simulink model "VSG"  (R2022a)
settings: Solver=ode23t  StartTime=0.0  StopTime=3  RelTol=1e-3
values from neighbouring files (symbols this model uses):
  C = 5600e-6    (= 0.0056)    [param.m]
  Cf = 35e-6    (= 3.5e-05)    [param.m]
  D = 3.24e4/w0    (= 103.132403124)    [param.m]
  E0 = 311    [param.m]
  fn = 50    [param.m]
  Ib = Sb/(sqrt(3)*Ub)    [param.m]
  J = 3.36    [param.m]
  Kf = 0.95e4/w0    (= 30.2394391875)    [param.m]
  Ki = 0.5*sqrt(3)*Sb/Ub    [param.m]
  Kq = (2500*6000)/(800e3*sqrt(3))    [param.m]
  L = 3e-3    (= 0.003)    [param.m]
  Pref = 170e3    (= 170000)    [param.m]
  R = 0.5    [param.m]
  Rc = 1e-3    (= 0.001)    [param.m]
  Rf = 0.05    [param.m]
  Sb = 800e3    (= 800000)    [param.m]
  Ts = 1/20e3    (= 5e-05)    [param.m]
  Ub = 6e3    (= 6000)    [param.m]
  Un = 380    [param.m]
  w0 = 2*pi*fn    (= 314.159265359)    [param.m]
libraries: spsIGBTDiodeLib x14, spsSeriesRLCBranchLib x9, slpidlib x7, spsDiodeLib x6, spsVoltageMeasurementLib x6, spsabctodq0Lib x4, spsThreePhaseVIMeasurementLib x3, eePowerMeasurement x2, simulink x2, spsDCVoltageSourceLib x1, spsGroundLib x1, spsPower3phInstantaneousLib x1
(part 1 of 2)
settings Model: Creator=Ziang Liu  LastModifiedBy=Ziang Liu

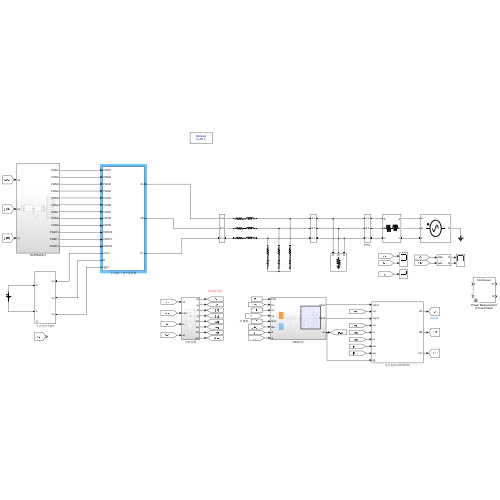
[thumbnail: Simulink's stored preview of the top-level diagram]
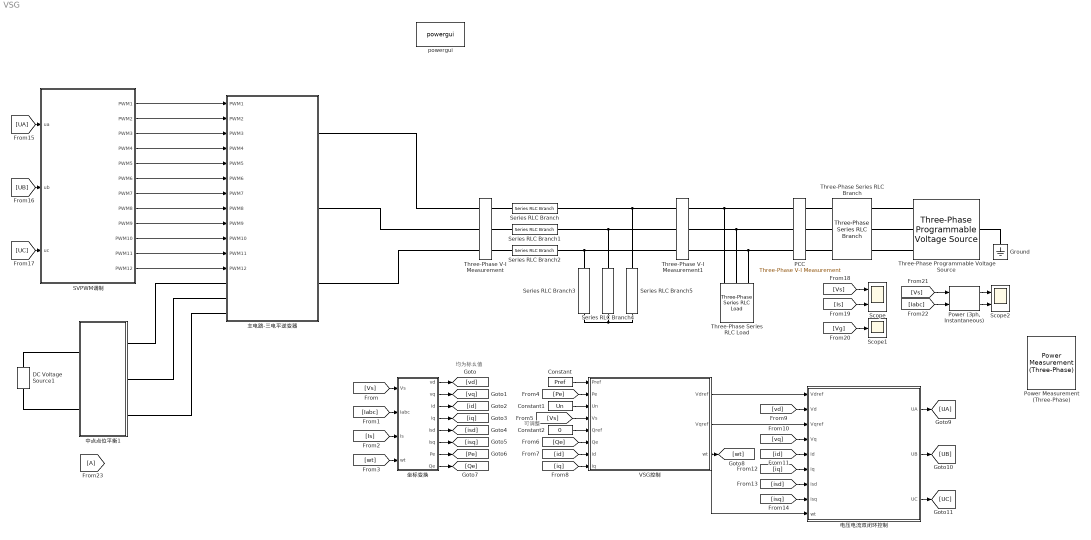
== system VSG ==
  note: 可调整
  note: 均为标幺值
  Constant : Constant  Value=Pref
  Constant1 : Constant  Value=Un
  Constant2 : Constant  Value=0
  DC Voltage Source1 : spsDCVoltageSourceLib/DC Voltage Source  Amplitude=1000  Measurements=None
  From23 : From
  Ground : spsGroundLib/Ground  LConnTagsString=a
  PCC : spsThreePhaseVIMeasurementLib/Three-Phase V-I Measurement  VoltageMeasurement=phase-to-ground  SetLabelV=on  LabelV=Vg  Vpu=off  VpuLL=off  CurrentMeasurement=no  SetLabelI=off  LabelI=Is  Ipu=off  Pbase=100e6  Vbase=500e3  OutputType=Complex  PhasorSimulation=off  PSBequivalent=0
  "Power (3ph, Instantaneous)" : spsPower3phInstantaneousLib/Power (3ph, Instantaneous)
  Power Measurement (Three-Phase) : eePowerMeasurement/Power Measurement (Three-Phase)  LabelModeActiveChoice=Continuous  F=60  K=[0 1 2 3]  Seq=Positive  Ts=0
      settings: SourceProductBaseCode=PS
  SVPWM调制 : Subsystem
  Scope : Scope  NumInputPorts=2
  Scope1 : Scope
  Scope2 : Scope  NumInputPorts=2
  Series RLC Branch : spsSeriesRLCBranchLib/Series RLC Branch  LConnTagsString=__new0  RConnTagsString=__new0  BranchType=RL  Resistance=Rf  Inductance=L  SetiL0=off  InitialCurrent=0  Capacitance=1e-6  Setx0=off  InitialVoltage=0  Measurements=None
  Series RLC Branch1 : spsSeriesRLCBranchLib/Series RLC Branch  LConnTagsString=__new0  RConnTagsString=__new0  BranchType=RL  Resistance=Rf  Inductance=L  SetiL0=off  InitialCurrent=0  Capacitance=1e-6  Setx0=off  InitialVoltage=0  Measurements=None
  Series RLC Branch2 : spsSeriesRLCBranchLib/Series RLC Branch  LConnTagsString=__new0  RConnTagsString=__new0  BranchType=RL  Resistance=Rf  Inductance=L  SetiL0=off  InitialCurrent=0  Capacitance=1e-6  Setx0=off  InitialVoltage=0  Measurements=None
  Series RLC Branch3 : spsSeriesRLCBranchLib/Series RLC Branch  LConnTagsString=__new0  RConnTagsString=__new0  BranchType=RC  Resistance=R  Inductance=L  SetiL0=off  InitialCurrent=0  Capacitance=Cf  Setx0=off  InitialVoltage=0  Measurements=None
  Series RLC Branch4 : spsSeriesRLCBranchLib/Series RLC Branch  LConnTagsString=__new0  RConnTagsString=__new0  BranchType=RC  Resistance=R  Inductance=L  SetiL0=off  InitialCurrent=0  Capacitance=Cf  Setx0=off  InitialVoltage=0  Measurements=None
  Series RLC Branch5 : spsSeriesRLCBranchLib/Series RLC Branch  LConnTagsString=__new0  RConnTagsString=__new0  BranchType=RC  Resistance=R  Inductance=L  SetiL0=off  InitialCurrent=0  Capacitance=Cf  Setx0=off  InitialVoltage=0  Measurements=None
  Three-Phase Programmable Voltage Source : spsThreePhaseProgrammableVoltageSourceLib/Three-Phase Programmable Voltage Source  PositiveSequence="[380  0 50]"  VariationEntity=Frequency  VariationType=Table of time-amplitude pairs  VariationTypeAlt=Step  VariationStep=-0.2  VariationRate=10  VariationMagnitude=0.3  VariationFrequency=2  VariationTiming=[1 2]  VariationPhaseA=off  Amplitudes=[1 0.8 1.2 1.0]  TimeValues=[0 0.1 0.15 0.2]  HarmonicGeneration=off  HarmonicA=[3 0.2 -25 0]  HarmonicB=[2 0.15 35 2]  Timing="[0.05  3]"  BusType=swing  Pref=0  Qref=0  Qmin=-inf  Qmax=inf
  Three-Phase Series RLC Branch : spsThreePhaseSeriesRLCBranchLib/Three-Phase Series RLC Branch  LConnTagsString=A|B|C  RConnTagsString=A|B|C  BranchType=RL  Resistance=0.06  Inductance=1.35e-3  Capacitance=1e-6  Measurements=None
  Three-Phase Series RLC Load : spsThreePhaseSeriesRLCLoadLib/Three-Phase Series RLC Load  LConnTagsString=A|B|C  Configuration=Y (grounded)  NominalVoltage=380  Vabc=[1e3 1e3 1e3]  Vabcp=[1e3 1e3 1e3]  NominalFrequency=50  UnbalancedPower=off  ActivePower=120e3  InductivePower=0  CapacitivePower=0  Pabc=[10e3 9e3 11e3]  QLabc=[100 90 110]  QCabc=[100 90 110]  Pabcp=[10e3 9e3 11e3]  QLabcp=[100 90 110]  QCabcp=[100 90 110]  Measurements=None  LoadType=constant Z
  Three-Phase V-I Measurement : spsThreePhaseVIMeasurementLib/Three-Phase V-I Measurement  VoltageMeasurement=no  SetLabelV=off  LabelV=Vabc  Vpu=off  VpuLL=off  CurrentMeasurement=yes  SetLabelI=on  LabelI=Iabc  Ipu=off  Pbase=100e6  Vbase=500e3  OutputType=Complex  PhasorSimulation=off  PSBequivalent=0
  Three-Phase V-I Measurement1 : spsThreePhaseVIMeasurementLib/Three-Phase V-I Measurement  VoltageMeasurement=phase-to-ground  SetLabelV=on  LabelV=Vs  Vpu=off  VpuLL=off  CurrentMeasurement=yes  SetLabelI=on  LabelI=Is  Ipu=off  Pbase=100e6  Vbase=500e3  OutputType=Complex  PhasorSimulation=off  PSBequivalent=0
  VSG控制 : Subsystem
  powergui : spspowerguiLib/powergui  Priority=1  SimulationMode=Discrete  SampleTime=1e-6  frequency=60  Iterations=50  frequencyindice=50  Pbase=100e6  ErrMax=1e-4  UnitsV=kV  UnitsW=MW  buscounter=0  FunctionMessages=off  echomessages=off  EnableUseOfTLC=off  CurrentSourceSwitches=off  DisableSnubberDevices=off  DisableRonSwitches=off  DisableVfSwitches=off  DisplayEquations=off  AutomaticDiscreteSolvers=off  SolverType=Tustin/Backward Euler (TBE)  Interpol=off  ExternalGateDelay=off  methode=off  Ts=100  x0status=blocks  SPID=on  SwTol=0  HookPort=off  NonlinearTolerance=1e-4  nMaxIteration=100  ContinueOnMaxIteration=off  RestoreLinks=warning  ResistiveCurrentMeasurement=off  Frange=[0:2:500]  Ylog=off  Xlog=on  ShowGrid=off  save=off  variable=ZData  structure=0  ZoomFFT=off  StartTime=0.0  cycles=1  DisplayStyle=1  fundamental=60  FreqAxis=off  MaxFrequency=1000  frequencyindicesteady=1  RmsSteady=1  display=off
  中点点位平衡1 : Subsystem  mask{Ln=2e-3, Kp1=20.73, Ki1=4.2, Kp2=5.5, Ki2=2.7}
      mask prompts: Ln "平衡电感Ln："; Kp1 "电压外环Kp1："; Ki1 "电压外环Ki1："; Kp2 "电流内环Kp2："; Ki2 "电流内环Ki2"
      mask DialogControl ParameterGroupVar Prompt: 参数
  主电路-三电平逆变器 : Subsystem  mask{Rc=1e-3, C=5600e-6}
      mask prompts: Rc "电容等效电阻Rc"; C "直流电容C:"
      mask DialogControl ParameterGroupVar Prompt: 参数
  坐标变换 : Subsystem
  电压电流双闭环控制 : Subsystem  mask{Kpu=6, Kiu=153.33, Kpi=4.2, Kii=0.323, wC=2*pi*fn*Cf*(Sb/(Ub^2)), wL=2*pi*fn*L*(Sb/(Ub^2))}
      mask prompts: Kpu "电压环比例系数Kpu:"; Kiu "电压环积分系数Kiu:"; Kpi "电流环比例系数Kpi:"; Kii "电流环v积分系数Kii:"; wC "耦合电容wC:"; wL "耦合电感wL:"
      mask DialogControl ParameterGroupVar Prompt: 参数
  wires:
  [Vs] -> 坐标变换/1(Vs)
  [Iabc] -> 坐标变换/2(Iabc)
  [Is] -> 坐标变换/3(Is)
  [wt] -> 坐标变换/4(wt)
  坐标变换/1(vd) -> [vd]
  坐标变换/2(vq) -> [vq]
  坐标变换/3(id) -> [id]
  坐标变换/4(iq) -> [iq]
  坐标变换/5(isd) -> [isd]
  坐标变换/7(Pe) -> [Pe]
  坐标变换/8(Qe) -> [Qe]
  坐标变换/6(isq) -> [isq]
  Constant/1 -> VSG控制/1(Pref)
  [Pe] -> VSG控制/2(Pe)
  Constant1/1 -> VSG控制/3(Un)
  [Vs] -> VSG控制/4(Vs)
  Constant2/1 -> VSG控制/5(Qref)
  [Qe] -> VSG控制/6(Qe)
  [id] -> VSG控制/7(id)
  [iq] -> VSG控制/8(iq)
  VSG控制/3(wt) -> 电压电流双闭环控制/9(wt), [wt]
  VSG控制/1(Vdref) -> 电压电流双闭环控制/1(Vdref)
  VSG控制/2(Vqref) -> 电压电流双闭环控制/3(Vqref)
  [vd] -> 电压电流双闭环控制/2(Vd)
  [vq] -> 电压电流双闭环控制/4(Vq)
  [id] -> 电压电流双闭环控制/5(id)
  [iq] -> 电压电流双闭环控制/6(iq)
  [isd] -> 电压电流双闭环控制/7(isd)
  [isq] -> 电压电流双闭环控制/8(isq)
  SVPWM调制/12(PWM12) -> 主电路-三电平逆变器/12(PWM12)
  SVPWM调制/8(PWM8) -> 主电路-三电平逆变器/8(PWM8)
  SVPWM调制/9(PWM9) -> 主电路-三电平逆变器/9(PWM9)
  SVPWM调制/6(PWM6) -> 主电路-三电平逆变器/6(PWM6)
  SVPWM调制/11(PWM11) -> 主电路-三电平逆变器/11(PWM11)
  SVPWM调制/10(PWM10) -> 主电路-三电平逆变器/10(PWM10)
  SVPWM调制/7(PWM7) -> 主电路-三电平逆变器/7(PWM7)
  SVPWM调制/2(PWM2) -> 主电路-三电平逆变器/2(PWM2)
  SVPWM调制/4(PWM4) -> 主电路-三电平逆变器/4(PWM4)
  SVPWM调制/5(PWM5) -> 主电路-三电平逆变器/5(PWM5)
  SVPWM调制/3(PWM3) -> 主电路-三电平逆变器/3(PWM3)
  SVPWM调制/1(PWM1) -> 主电路-三电平逆变器/1(PWM1)
  电压电流双闭环控制/1(UA) -> [UA]
  电压电流双闭环控制/2(UB) -> [UB]
  电压电流双闭环控制/3(UC) -> [UC]
  [UA] -> SVPWM调制/1(ua)
  [UB] -> SVPWM调制/2(ub)
  [UC] -> SVPWM调制/3(uc)
  [Vs] -> Scope/1
  [Is] -> Scope/2
  [Vg] -> Scope1/1
  [Vs] -> "Power (3ph, Instantaneous)"/1
  [Iabc] -> "Power (3ph, Instantaneous)"/2
  "Power (3ph, Instantaneous)"/1 -> Scope2/1
  "Power (3ph, Instantaneous)"/2 -> Scope2/2
  connections:
  Three-Phase V-I Measurement/RConn3 -- Series RLC Branch2/LConn1
  Three-Phase V-I Measurement/RConn2 -- Series RLC Branch1/LConn1
  Series RLC Branch/LConn1 -- Three-Phase V-I Measurement/RConn1
  Series RLC Branch3/RConn1 -- Series RLC Branch4/RConn1 -- Series RLC Branch5/RConn1
  Series RLC Branch2/RConn1 -- Three-Phase V-I Measurement1/LConn3 -- Series RLC Branch3/LConn1
  Series RLC Branch1/RConn1 -- Three-Phase V-I Measurement1/LConn2 -- Series RLC Branch4/LConn1
  Series RLC Branch/RConn1 -- Three-Phase V-I Measurement1/LConn1 -- Series RLC Branch5/LConn1
  Three-Phase V-I Measurement1/RConn3 -- Three-Phase Series RLC Load/LConn3 -- PCC/LConn3
  PCC/LConn2 -- Three-Phase Series RLC Load/LConn2 -- Three-Phase V-I Measurement1/RConn2
  Three-Phase V-I Measurement1/RConn1 -- Three-Phase Series RLC Load/LConn1 -- PCC/LConn1
  Three-Phase Series RLC Branch/LConn1 -- PCC/RConn1
  Three-Phase Series RLC Branch/LConn2 -- PCC/RConn2
  Three-Phase Series RLC Branch/LConn3 -- PCC/RConn3
  Three-Phase Programmable Voltage Source/RConn1 -- Three-Phase Series RLC Branch/RConn1
  Three-Phase Programmable Voltage Source/RConn2 -- Three-Phase Series RLC Branch/RConn2
  Three-Phase Programmable Voltage Source/RConn3 -- Three-Phase Series RLC Branch/RConn3
  Ground/LConn1 -- Three-Phase Programmable Voltage Source/LConn1
  DC Voltage Source1/RConn1 -- 中点点位平衡1/LConn1
  DC Voltage Source1/LConn1 -- 中点点位平衡1/LConn2
  中点点位平衡1/RConn2 -- 主电路-三电平逆变器/LConn2
  中点点位平衡1/RConn1 -- 主电路-三电平逆变器/LConn1
  中点点位平衡1/RConn3 -- 主电路-三电平逆变器/LConn3
  Three-Phase V-I Measurement/LConn3 -- 主电路-三电平逆变器/RConn3
  Three-Phase V-I Measurement/LConn2 -- 主电路-三电平逆变器/RConn2
  Three-Phase V-I Measurement/LConn1 -- 主电路-三电平逆变器/RConn1

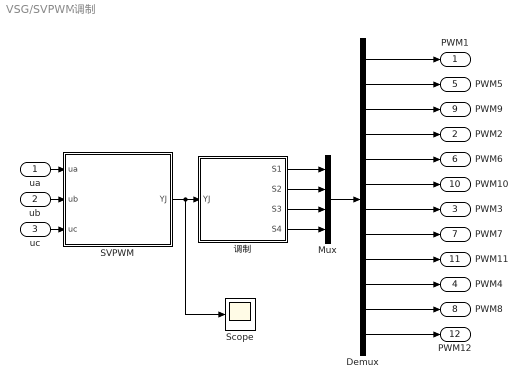
== system VSG/SVPWM调制 ==
  ua : Inport
  ub : Inport  Port=2
  uc : Inport  Port=3
  Demux : Demux  Outputs=12
  Mux : Mux
  SVPWM : Subsystem
  Scope : Scope
  调制 : Subsystem
  PWM1 : Outport
  PWM2 : Outport  Port=2
  PWM3 : Outport  Port=3
  PWM4 : Outport  Port=4
  PWM5 : Outport  Port=5
  PWM6 : Outport  Port=6
  PWM7 : Outport  Port=7
  PWM8 : Outport  Port=8
  PWM9 : Outport  Port=9
  PWM10 : Outport  Port=10
  PWM11 : Outport  Port=11
  PWM12 : Outport  Port=12
  wires:
  Demux/4 -> PWM2/1
  Demux/9 -> PWM11/1
  SVPWM/1(YJ) -> Scope/1, 调制/1(YJ)
  ub/1 -> SVPWM/2(ub)
  Mux/1 -> Demux/1
  Demux/10 -> PWM4/1
  Demux/2 -> PWM5/1
  Demux/1 -> PWM1/1
  Demux/3 -> PWM9/1
  Demux/8 -> PWM7/1
  ua/1 -> SVPWM/1(ua)
  Demux/11 -> PWM8/1
  Demux/5 -> PWM6/1
  调制/4(S4) -> Mux/4
  调制/1(S1) -> Mux/1
  Demux/6 -> PWM10/1
  Demux/12 -> PWM12/1
  uc/1 -> SVPWM/3(uc)
  调制/3(S3) -> Mux/3
  调制/2(S2) -> Mux/2
  Demux/7 -> PWM3/1

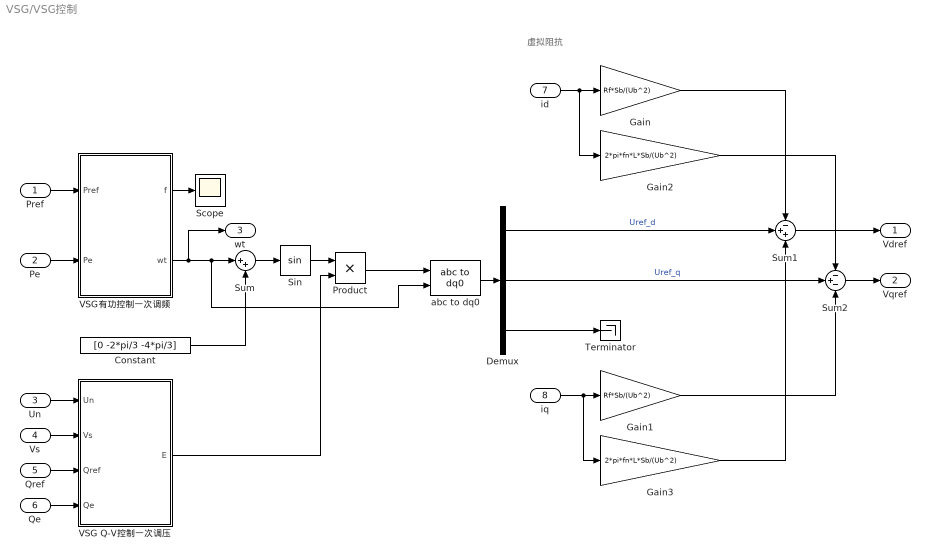
== system VSG/VSG控制 ==
  note: 虚拟阻抗
  Pref : Inport
  Pe : Inport  Port=2
  Un : Inport  Port=3
  Vs : Inport  Port=4
  Qref : Inport  Port=5
  Qe : Inport  Port=6
  id : Inport  Port=7
  iq : Inport  Port=8
  Constant : Constant  Value=[0 -2*pi/3 -4*pi/3]
  Demux : Demux  Outputs=3
  Gain : Gain  Gain=Rf*Sb/(Ub^2)
  Gain1 : Gain  Gain=Rf*Sb/(Ub^2)
  Gain2 : Gain  Gain=2*pi*fn*L*Sb/(Ub^2)
  Gain3 : Gain  Gain=2*pi*fn*L*Sb/(Ub^2)
  Product : Product
  Scope : Scope
  Sin : Trigonometry
  Sum : Sum  Inputs=|++
  Sum1 : Sum  Inputs=-++
  Sum2 : Sum  Inputs=-+-
  Terminator : Terminator
  VSG Q-V控制一次调压 : Subsystem
  VSG有功控制一次调频 : Subsystem
  abc to dq0 : spsabctodq0Lib/abc to dq0  Alignment=90 degrees behind phase A axis
  Vdref : Outport
  Vqref : Outport  Port=2
  wt : Outport  Port=3
  wires:
  Gain/1 -> Sum1/1
  Vs/1 -> VSG Q-V控制一次调压/2(Vs)
  Gain2/1 -> Sum2/1
  Sum1/1 -> Vdref/1
  iq/1 -> Gain1/1, Gain3/1
  Gain1/1 -> Sum2/3
  VSG有功控制一次调频/1(f) -> Scope/1
  id/1 -> Gain2/1, Gain/1
  Sin/1 -> Product/1
  Pe/1 -> VSG有功控制一次调频/2(Pe)
  Product/1 -> abc to dq0/1
  Sum2/1 -> Vqref/1
  Sum/1 -> Sin/1
  Qe/1 -> VSG Q-V控制一次调压/4(Qe)
  VSG有功控制一次调频/2(wt) -> wt/1, abc to dq0/2, Sum/1
  Constant/1 -> Sum/2
  Qref/1 -> VSG Q-V控制一次调压/3(Qref)
  Gain3/1 -> Sum1/3
  Un/1 -> VSG Q-V控制一次调压/1(Un)
  Pref/1 -> VSG有功控制一次调频/1(Pref)
  Demux/1 -> Sum1/2  "Uref_d"
  VSG Q-V控制一次调压/1(E) -> Product/2
  abc to dq0/1 -> Demux/1
  Demux/2 -> Sum2/2  "Uref_q"
  Demux/3 -> Terminator/1

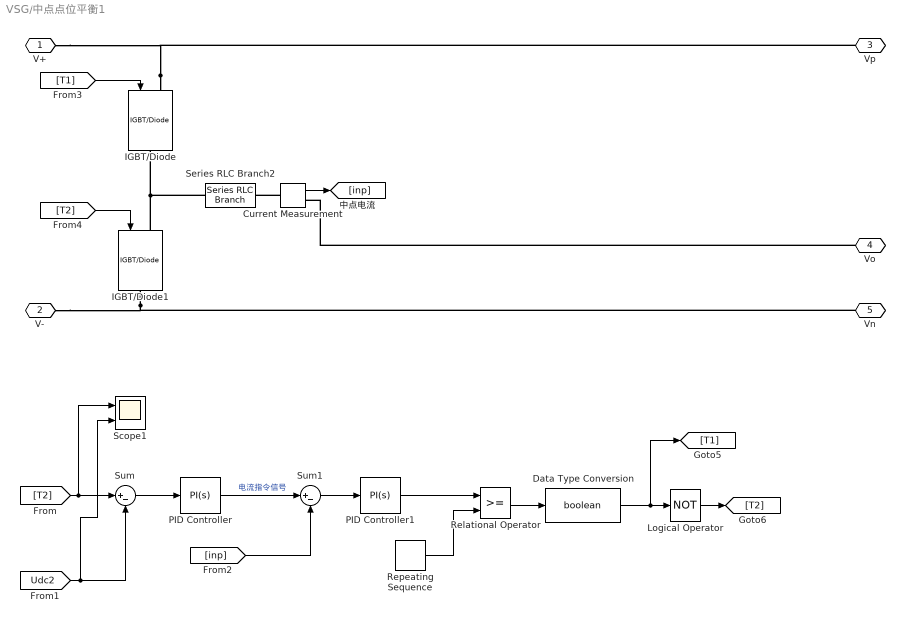
== system VSG/中点点位平衡1 ==
  Current Measurement : spsCurrentMeasurementLib/Current Measurement  PhasorSimulation=off  OutputType=Complex  PSBequivalent=0
  Data Type Conversion : DataTypeConversion  OutMin=[0]  OutMax=[1]  OutDataTypeStr=boolean  SaturateOnIntegerOverflow=off  RndMeth=Floor
  IGBT/Diode : spsIGBTDiodeLib/IGBT//Diode  Ron=1e-3  Rs=1e5  Cs=inf  Measurements=off
  IGBT/Diode1 : spsIGBTDiodeLib/IGBT//Diode  Ron=1e-3  Rs=1e5  Cs=inf  Measurements=off
  Logical Operator : Logic  Operator=NOT  AllPortsSameDT=off  OutDataTypeStr=boolean
  PID Controller : slpidlib/PID Controller  Controller=PI  Form=Parallel  TimeDomain=Continuous-time  UseExternalTs=off  SampleTime=-1  IntegratorMethod=Forward Euler  FilterMethod=Forward Euler  ControllerParametersSource=internal  P=Kp1  I=Ki1  UseKiTs=off  D=0  N=100  UseFilter=on  TunerSelectOption=Transfer Function Based (PID Tuner App)  InitialConditionSource=internal  InitialConditionForIntegrator=0  InitialConditionForFilter=0  DifferentiatorICPrevScaledInput=0  ExternalReset=none  TrackingMode=off  Kt=1  LimitOutput=off  SatLimitsSource=internal  UpperSaturationLimit=inf  LowerSaturationLimit=-inf  LinearizeAsGain=on  AntiWindupMode=none  Kb=1  POutMin=[]  POutMax=[]  IOutMin=[]  IOutMax=[]  DOutMin=[]  DOutMax=[]  NOutMin=[]  NOutMax=[]  SumOutMin=[]  SumOutMax=[]  SaturationOutMin=[]  SaturationOutMax=[]  PParamMin=[]  PParamMax=[]  IParamMin=[]  IParamMax=[]  DParamMin=[]  DParamMax=[]  NParamMin=[]  NParamMax=[]  KbParamMin=[]  KbParamMax=[]  KtParamMin=[]  KtParamMax=[]  KbOutMin=[]  KbOutMax=[]  KtOutMin=[]  KtOutMax=[]  IntegratorOutMin=[]  IntegratorOutMax=[]  FilterOutMin=[]  FilterOutMax=[]  SumI1OutMin=[]  SumI1OutMax=[]  SumI2OutMin=[]  SumI2OutMax=[]  SumI3OutMin=[]  SumI3OutMax=[]  SumI4OutMin=[]  SumI4OutMax=[]  SumDOutMin=[]  SumDOutMax=[]  DifferentiatorOutMin=[]  DifferentiatorOutMax=[]  FilterDiffOutCoefMin=[]  FilterDiffOutCoefMax=[]  ReciprocalOutMin=[]  ReciprocalOutMax=[]  SumDenOutMin=[]  SumDenOutMax=[]  SumNumOutMin=[]  SumNumOutMax=[]  DivideOutMin=[]  DivideOutMax=[]  UdiffTsProdOutMin=[]  UdiffTsProdOutMax=[]  NTsProdOutMin=[]  NTsProdOutMax=[]  UintegralTsProdOutMin=[]  UintegralTsProdOutMax=[]  UngainTsProdOutMin=[]  UngainTsProdOutMax=[]  IntegratorContinuousStateAttributes=''  IntegratorStateMustResolveToSignalObject=off  IntegratorRTWStateStorageClass=Auto  FilterContinuousStateAttributes=''  FilterStateMustResolveToSignalObject=off  FilterRTWStateStorageClass=Auto  ParallelPVariant=InternalParameters  IdealPVariant=Disabled  IVariant=InternalParameters  DVariant=Disabled  IntegratorVariant=Continuous  SatVariant=Disabled  AWVariant=Passthrough  PCopyVariant=Disabled  TRVariant=Disabled  FdbkBlocksVariant=Forward  IdealPFdbkVariant=Disabled  SatFdbkVariant=Disabled  DerivativeFilterVariant=Disabled  NVariant=Disabled  NCopyVariant=Disabled_SignalSpec  FilterICVariant=Disabled  IntegratorICVariant=InternalICs  ExternalResetVariant=Disabled  TRSumVariant=Passthrough  SumFdbkVariant=Disabled  SumVariant=Sum_PI  TsampFilterVariant=InternalTs  TsampNgainVariant=Passthrough  TsampIntegralVariant=Passthrough  ExternalSaturationOutDataTypeStr=Inherit: Same as second input  aMode=0
  PID Controller1 : slpidlib/PID Controller  Controller=PI  Form=Parallel  TimeDomain=Continuous-time  UseExternalTs=off  SampleTime=-1  IntegratorMethod=Forward Euler  FilterMethod=Forward Euler  ControllerParametersSource=internal  P=Kp2  I=Ki2  UseKiTs=off  D=0  N=100  UseFilter=on  TunerSelectOption=Transfer Function Based (PID Tuner App)  InitialConditionSource=internal  InitialConditionForIntegrator=0  InitialConditionForFilter=0  DifferentiatorICPrevScaledInput=0  ExternalReset=none  TrackingMode=off  Kt=1  LimitOutput=off  SatLimitsSource=internal  UpperSaturationLimit=inf  LowerSaturationLimit=-inf  LinearizeAsGain=on  AntiWindupMode=none  Kb=1  POutMin=[]  POutMax=[]  IOutMin=[]  IOutMax=[]  DOutMin=[]  DOutMax=[]  NOutMin=[]  NOutMax=[]  SumOutMin=[]  SumOutMax=[]  SaturationOutMin=[]  SaturationOutMax=[]  PParamMin=[]  PParamMax=[]  IParamMin=[]  IParamMax=[]  DParamMin=[]  DParamMax=[]  NParamMin=[]  NParamMax=[]  KbParamMin=[]  KbParamMax=[]  KtParamMin=[]  KtParamMax=[]  KbOutMin=[]  KbOutMax=[]  KtOutMin=[]  KtOutMax=[]  IntegratorOutMin=[]  IntegratorOutMax=[]  FilterOutMin=[]  FilterOutMax=[]  SumI1OutMin=[]  SumI1OutMax=[]  SumI2OutMin=[]  SumI2OutMax=[]  SumI3OutMin=[]  SumI3OutMax=[]  SumI4OutMin=[]  SumI4OutMax=[]  SumDOutMin=[]  SumDOutMax=[]  DifferentiatorOutMin=[]  DifferentiatorOutMax=[]  FilterDiffOutCoefMin=[]  FilterDiffOutCoefMax=[]  ReciprocalOutMin=[]  ReciprocalOutMax=[]  SumDenOutMin=[]  SumDenOutMax=[]  SumNumOutMin=[]  SumNumOutMax=[]  DivideOutMin=[]  DivideOutMax=[]  UdiffTsProdOutMin=[]  UdiffTsProdOutMax=[]  NTsProdOutMin=[]  NTsProdOutMax=[]  UintegralTsProdOutMin=[]  UintegralTsProdOutMax=[]  UngainTsProdOutMin=[]  UngainTsProdOutMax=[]  IntegratorContinuousStateAttributes=''  IntegratorStateMustResolveToSignalObject=off  IntegratorRTWStateStorageClass=Auto  FilterContinuousStateAttributes=''  FilterStateMustResolveToSignalObject=off  FilterRTWStateStorageClass=Auto  ParallelPVariant=InternalParameters  IdealPVariant=Disabled  IVariant=InternalParameters  DVariant=Disabled  IntegratorVariant=Continuous  SatVariant=Disabled  AWVariant=Passthrough  PCopyVariant=Disabled  TRVariant=Disabled  FdbkBlocksVariant=Forward  IdealPFdbkVariant=Disabled  SatFdbkVariant=Disabled  DerivativeFilterVariant=Disabled  NVariant=Disabled  NCopyVariant=Disabled_SignalSpec  FilterICVariant=Disabled  IntegratorICVariant=InternalICs  ExternalResetVariant=Disabled  TRSumVariant=Passthrough  SumFdbkVariant=Disabled  SumVariant=Sum_PI  TsampFilterVariant=InternalTs  TsampNgainVariant=Passthrough  TsampIntegralVariant=Passthrough  ExternalSaturationOutDataTypeStr=Inherit: Same as second input  aMode=0
  Relational Operator : RelationalOperator  OutDataTypeStr=boolean  RndMeth=Simplest  InputSameDT=off
  Repeating Sequence : simulink/Sources/Repeating Sequence  rep_seq_t=[0 0.5*Ts Ts]  rep_seq_y=[-1 1 -1]
  Scope1 : Scope  NumInputPorts=2
  Series RLC Branch2 : spsSeriesRLCBranchLib/Series RLC Branch  LConnTagsString=__new0  RConnTagsString=__new0  BranchType=L  Resistance=Rc  Inductance=Ln  SetiL0=off  InitialCurrent=0  Capacitance=C  Setx0=off  InitialVoltage=0  Measurements=None
  Sum : Sum  Inputs=|+-
  Sum1 : Sum  Inputs=|+-
  V+ : PMIOPort  Side=Left
  V- : PMIOPort  Port=2  Side=Left
  Vp : PMIOPort  Port=3  Side=Right
  Vo : PMIOPort  Port=4  Side=Right
  Vn : PMIOPort  Port=5  Side=Right
  wires:
  [T2] -> IGBT/Diode1/1
  Relational Operator/1 -> Data Type Conversion/1
  [Udc2] -> Scope1/2, Sum/2
  Data Type Conversion/1 -> Logical Operator/1, [T1]
  Sum1/1 -> PID Controller1/1
  [T2] -> Scope1/1, Sum/1
  Current Measurement/1 -> [inp]
  Sum/1 -> PID Controller/1
  [inp] -> Sum1/2
  Logical Operator/1 -> [T2]
  PID Controller/1 -> Sum1/1  "电流指令信号"
  PID Controller1/1 -> Relational Operator/1
  [T1] -> IGBT/Diode/1
  Repeating Sequence/1 -> Relational Operator/2
  connections:
  Current Measurement/LConn1 -- Series RLC Branch2/LConn1
  IGBT/Diode1/RConn1 -- Vn/RConn1 -- V-/RConn1
  IGBT/Diode/LConn1 -- Vp/RConn1 -- V+/RConn1
  IGBT/Diode1/LConn1 -- Series RLC Branch2/RConn1 -- IGBT/Diode/RConn1
  Vo/RConn1 -- Current Measurement/RConn1

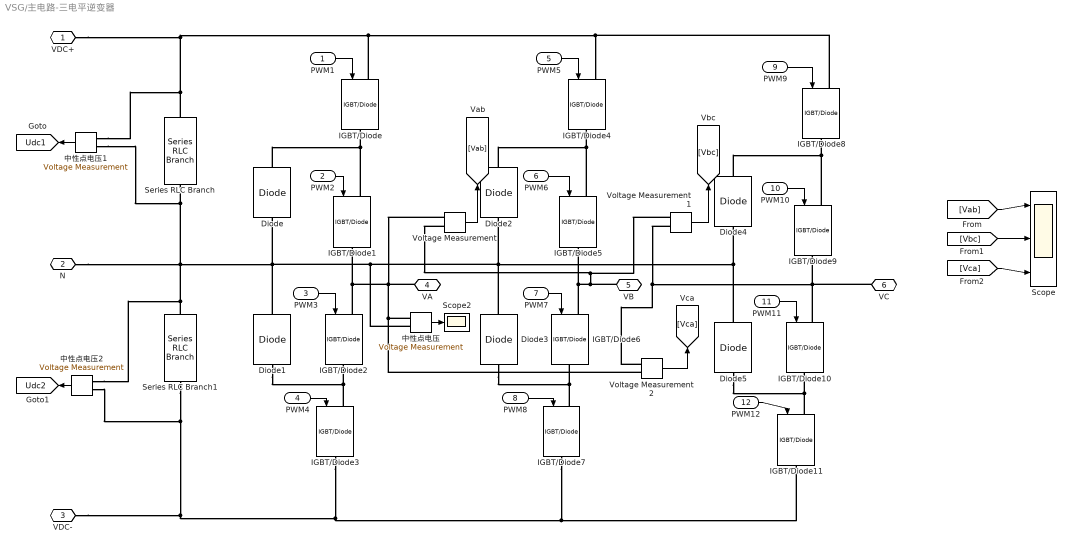
== system VSG/主电路-三电平逆变器 ==
  PWM1 : Inport
  PWM2 : Inport  Port=2
  PWM3 : Inport  Port=3
  PWM4 : Inport  Port=4
  PWM5 : Inport  Port=5
  PWM6 : Inport  Port=6
  PWM7 : Inport  Port=7
  PWM8 : Inport  Port=8
  PWM9 : Inport  Port=9
  PWM10 : Inport  Port=10
  PWM11 : Inport  Port=11
  PWM12 : Inport  Port=12
  Diode{,1..5} (6 alike) : spsDiodeLib/Diode  Ron=0.001  Lon=0  Vf=0.8  IC=0  UseSnubber=0  Rs=500  Cs=250e-9  Measurements=off
  IGBT/Diode{,1..11} (12 alike) : spsIGBTDiodeLib/IGBT//Diode  Ron=1e-3  Rs=1e5  Cs=inf  Measurements=off
  Scope : Scope  NumInputPorts=3
  Scope2 : Scope
  Series RLC Branch : spsSeriesRLCBranchLib/Series RLC Branch  LConnTagsString=__new0  RConnTagsString=__new0  BranchType=RC  Resistance=Rc  Inductance=1e-3  SetiL0=off  InitialCurrent=0  Capacitance=C  Setx0=off  InitialVoltage=0  Measurements=None
  Series RLC Branch1 : spsSeriesRLCBranchLib/Series RLC Branch  LConnTagsString=__new0  RConnTagsString=__new0  BranchType=RC  Resistance=Rc  Inductance=1e-3  SetiL0=off  InitialCurrent=0  Capacitance=C  Setx0=off  InitialVoltage=0  Measurements=None
  Voltage Measurement : spsVoltageMeasurementLib/Voltage Measurement  PhasorSimulation=off  OutputType=Complex  PSBequivalent=0
  Voltage Measurement1 : spsVoltageMeasurementLib/Voltage Measurement  PhasorSimulation=off  OutputType=Complex  PSBequivalent=0
  Voltage Measurement2 : spsVoltageMeasurementLib/Voltage Measurement  PhasorSimulation=off  OutputType=Complex  PSBequivalent=0
  中性点电压 : spsVoltageMeasurementLib/Voltage Measurement  PhasorSimulation=off  OutputType=Complex  PSBequivalent=0
  中性点电压1 : spsVoltageMeasurementLib/Voltage Measurement  PhasorSimulation=off  OutputType=Complex  PSBequivalent=0
  中性点电压2 : spsVoltageMeasurementLib/Voltage Measurement  PhasorSimulation=off  OutputType=Complex  PSBequivalent=0
  VDC+ : PMIOPort  Side=Left
  N : PMIOPort  Port=2  Side=Left
  VDC- : PMIOPort  Port=3  Side=Left
  VA : PMIOPort  Port=4  Side=Right
  VB : PMIOPort  Port=5  Side=Right
  VC : PMIOPort  Port=6  Side=Right
  tag scope: Udc1=global, Udc2=global
  wires:
  PWM8/1 -> IGBT/Diode7/1
  Voltage Measurement1/1 -> [Vbc]
  [Vbc] -> Scope/2
  PWM7/1 -> IGBT/Diode6/1
  PWM6/1 -> IGBT/Diode5/1
  PWM12/1 -> IGBT/Diode11/1
  PWM10/1 -> IGBT/Diode9/1
  PWM9/1 -> IGBT/Diode8/1
  PWM5/1 -> IGBT/Diode4/1
  PWM11/1 -> IGBT/Diode10/1
  PWM2/1 -> IGBT/Diode1/1
  中性点电压/1 -> Scope2/1
  PWM3/1 -> IGBT/Diode2/1
  Voltage Measurement2/1 -> [Vca]
  Voltage Measurement/1 -> [Vab]
  PWM1/1 -> IGBT/Diode/1
  PWM4/1 -> IGBT/Diode3/1
  [Vab] -> Scope/1
  [Vca] -> Scope/3
  中性点电压1/1 -> [Udc1]
  中性点电压2/1 -> [Udc2]
  connections:
  IGBT/Diode/LConn1 -- 中性点电压1/LConn1 -- Series RLC Branch/LConn1 -- VDC+/RConn1 -- IGBT/Diode4/LConn1 -- IGBT/Diode8/LConn1
  IGBT/Diode3/RConn1 -- Series RLC Branch1/RConn1 -- 中性点电压2/LConn2 -- VDC-/RConn1 -- IGBT/Diode7/RConn1 -- IGBT/Diode11/RConn1
  IGBT/Diode6/LConn1 -- VB/RConn1 -- Voltage Measurement1/LConn1 -- Voltage Measurement/LConn2 -- IGBT/Diode5/RConn1
  Series RLC Branch1/LConn1 -- Diode3/RConn1 -- Diode4/LConn1 -- Diode5/RConn1 -- Diode2/LConn1 -- 中性点电压/LConn2 -- Diode/LConn1 -- Diode1/RConn1 -- N/RConn1 -- 中性点电压1/LConn2 -- Series RLC Branch/RConn1 -- 中性点电压2/LConn1
  IGBT/Diode10/LConn1 -- VC/RConn1 -- Voltage Measurement2/LConn1 -- Voltage Measurement1/LConn2 -- IGBT/Diode9/RConn1
  IGBT/Diode2/LConn1 -- VA/RConn1 -- 中性点电压/LConn1 -- Voltage Measurement2/LConn2 -- Voltage Measurement/LConn1 -- IGBT/Diode1/RConn1
  Diode3/LConn1 -- IGBT/Diode7/LConn1 -- IGBT/Diode6/RConn1
  IGBT/Diode1/LConn1 -- Diode/RConn1 -- IGBT/Diode/RConn1
  IGBT/Diode5/LConn1 -- IGBT/Diode4/RConn1 -- Diode2/RConn1
  IGBT/Diode3/LConn1 -- Diode1/LConn1 -- IGBT/Diode2/RConn1
  IGBT/Diode8/RConn1 -- IGBT/Diode9/LConn1 -- Diode4/RConn1
  IGBT/Diode11/LConn1 -- Diode5/LConn1 -- IGBT/Diode10/RConn1

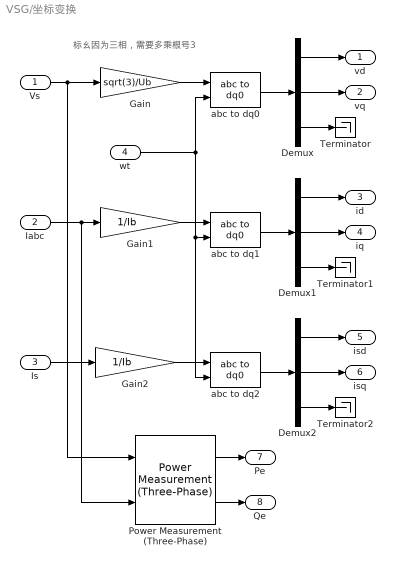
== system VSG/坐标变换 ==
  note: 标幺因为三相，需要多乘根号3
  Vs : Inport
  Iabc : Inport  Port=2
  Is : Inport  Port=3
  wt : Inport  Port=4
  Demux : Demux  Outputs=3
  Demux1 : Demux  Outputs=3
  Demux2 : Demux  Outputs=3
  Gain : Gain  Gain=sqrt(3)/Ub
  Gain1 : Gain  Gain=1/Ib
  Gain2 : Gain  Gain=1/Ib
  Power Measurement (Three-Phase) : eePowerMeasurement/Power Measurement (Three-Phase)  LabelModeActiveChoice=Continuous  F=50  K=[1]  Seq=Positive  Ts=0
      settings: SourceProductBaseCode=PS
  Terminator : Terminator
  Terminator1 : Terminator
  Terminator2 : Terminator
  abc to dq0 : spsabctodq0Lib/abc to dq0  Alignment=90 degrees behind phase A axis
  abc to dq1 : spsabctodq0Lib/abc to dq0  Alignment=90 degrees behind phase A axis
  abc to dq2 : spsabctodq0Lib/abc to dq0  Alignment=90 degrees behind phase A axis
  vd : Outport
  vq : Outport  Port=2
  id : Outport  Port=3
  iq : Outport  Port=4
  isd : Outport  Port=5
  isq : Outport  Port=6
  Pe : Outport  Port=7
  Qe : Outport  Port=8
  wires:
  abc to dq2/1 -> Demux2/1
  Vs/1 -> Power Measurement (Three-Phase)/1, Gain/1
  Gain1/1 -> abc to dq1/1
  Iabc/1 -> Power Measurement (Three-Phase)/2, Gain1/1
  abc to dq1/1 -> Demux1/1
  Demux/2 -> vq/1
  Gain2/1 -> abc to dq2/1
  Demux1/1 -> id/1
  Demux1/3 -> Terminator1/1
  Demux2/3 -> Terminator2/1
  Power Measurement (Three-Phase)/2 -> Qe/1
  wt/1 -> abc to dq0/2, abc to dq2/2, abc to dq1/2
  abc to dq0/1 -> Demux/1
  Demux/1 -> vd/1
  Demux/3 -> Terminator/1
  Demux1/2 -> iq/1
  Power Measurement (Three-Phase)/1 -> Pe/1
  Gain/1 -> abc to dq0/1
  Is/1 -> Gain2/1
  Demux2/1 -> isd/1
  Demux2/2 -> isq/1

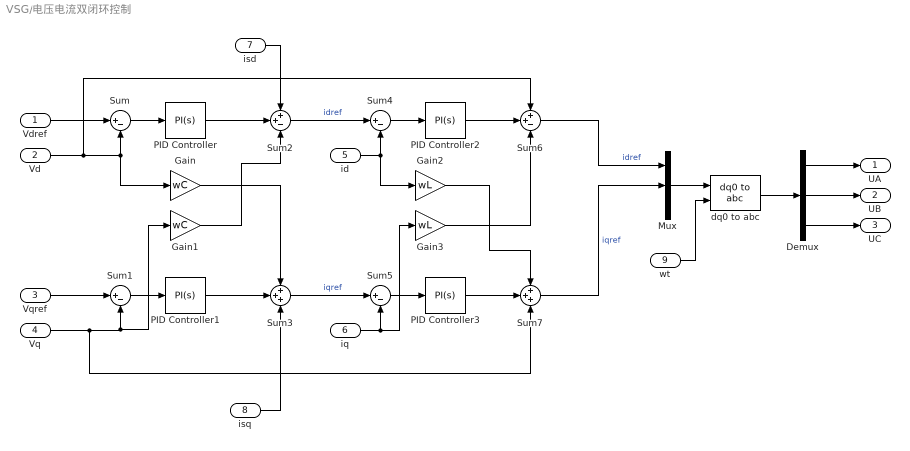
== system VSG/电压电流双闭环控制 ==
  Vdref : Inport
  Vd : Inport  Port=2
  Vqref : Inport  Port=3
  Vq : Inport  Port=4
  id : Inport  Port=5
  iq : Inport  Port=6
  isd : Inport  Port=7
  isq : Inport  Port=8
  wt : Inport  Port=9
  Demux : Demux  Outputs=3
  Gain : Gain  Gain=wC
  Gain1 : Gain  Gain=wC
  Gain2 : Gain  Gain=wL
  Gain3 : Gain  Gain=wL
  Mux : Mux  Inputs=3
  PID Controller : slpidlib/PID Controller  Controller=PI  Form=Parallel  TimeDomain=Continuous-time  UseExternalTs=off  SampleTime=-1  IntegratorMethod=Forward Euler  FilterMethod=Forward Euler  ControllerParametersSource=internal  P=Kpu  I=Kiu  UseKiTs=off  D=0  N=100  UseFilter=on  TunerSelectOption=Transfer Function Based (PID Tuner App)  InitialConditionSource=internal  InitialConditionForIntegrator=0  InitialConditionForFilter=0  DifferentiatorICPrevScaledInput=0  ExternalReset=none  TrackingMode=off  Kt=1  LimitOutput=off  SatLimitsSource=internal  UpperSaturationLimit=inf  LowerSaturationLimit=-inf  LinearizeAsGain=on  AntiWindupMode=none  Kb=1  POutMin=[]  POutMax=[]  IOutMin=[]  IOutMax=[]  DOutMin=[]  DOutMax=[]  NOutMin=[]  NOutMax=[]  SumOutMin=[]  SumOutMax=[]  SaturationOutMin=[]  SaturationOutMax=[]  PParamMin=[]  PParamMax=[]  IParamMin=[]  IParamMax=[]  DParamMin=[]  DParamMax=[]  NParamMin=[]  NParamMax=[]  KbParamMin=[]  KbParamMax=[]  KtParamMin=[]  KtParamMax=[]  KbOutMin=[]  KbOutMax=[]  KtOutMin=[]  KtOutMax=[]  IntegratorOutMin=[]  IntegratorOutMax=[]  FilterOutMin=[]  FilterOutMax=[]  SumI1OutMin=[]  SumI1OutMax=[]  SumI2OutMin=[]  SumI2OutMax=[]  SumI3OutMin=[]  SumI3OutMax=[]  SumI4OutMin=[]  SumI4OutMax=[]  SumDOutMin=[]  SumDOutMax=[]  DifferentiatorOutMin=[]  DifferentiatorOutMax=[]  FilterDiffOutCoefMin=[]  FilterDiffOutCoefMax=[]  ReciprocalOutMin=[]  ReciprocalOutMax=[]  SumDenOutMin=[]  SumDenOutMax=[]  SumNumOutMin=[]  SumNumOutMax=[]  DivideOutMin=[]  DivideOutMax=[]  UdiffTsProdOutMin=[]  UdiffTsProdOutMax=[]  NTsProdOutMin=[]  NTsProdOutMax=[]  UintegralTsProdOutMin=[]  UintegralTsProdOutMax=[]  UngainTsProdOutMin=[]  UngainTsProdOutMax=[]  IntegratorContinuousStateAttributes=''  IntegratorStateMustResolveToSignalObject=off  IntegratorRTWStateStorageClass=Auto  FilterContinuousStateAttributes=''  FilterStateMustResolveToSignalObject=off  FilterRTWStateStorageClass=Auto  ParallelPVariant=InternalParameters  IdealPVariant=Disabled  IVariant=InternalParameters  DVariant=Disabled  IntegratorVariant=Continuous  SatVariant=Disabled  AWVariant=Passthrough  PCopyVariant=Disabled  TRVariant=Disabled  FdbkBlocksVariant=Forward  IdealPFdbkVariant=Disabled  SatFdbkVariant=Disabled  DerivativeFilterVariant=Disabled  NVariant=Disabled  NCopyVariant=Disabled_SignalSpec  FilterICVariant=Disabled  IntegratorICVariant=InternalICs  ExternalResetVariant=Disabled  TRSumVariant=Passthrough  SumFdbkVariant=Disabled  SumVariant=Sum_PI  TsampFilterVariant=InternalTs  TsampNgainVariant=Passthrough  TsampIntegralVariant=Passthrough  ExternalSaturationOutDataTypeStr=Inherit: Same as second input  aMode=0
  PID Controller1 : slpidlib/PID Controller  Controller=PI  Form=Parallel  TimeDomain=Continuous-time  UseExternalTs=off  SampleTime=-1  IntegratorMethod=Forward Euler  FilterMethod=Forward Euler  ControllerParametersSource=internal  P=Kpu  I=Kiu  UseKiTs=off  D=0  N=100  UseFilter=on  TunerSelectOption=Transfer Function Based (PID Tuner App)  InitialConditionSource=internal  InitialConditionForIntegrator=0  InitialConditionForFilter=0  DifferentiatorICPrevScaledInput=0  ExternalReset=none  TrackingMode=off  Kt=1  LimitOutput=off  SatLimitsSource=internal  UpperSaturationLimit=inf  LowerSaturationLimit=-inf  LinearizeAsGain=on  AntiWindupMode=none  Kb=1  POutMin=[]  POutMax=[]  IOutMin=[]  IOutMax=[]  DOutMin=[]  DOutMax=[]  NOutMin=[]  NOutMax=[]  SumOutMin=[]  SumOutMax=[]  SaturationOutMin=[]  SaturationOutMax=[]  PParamMin=[]  PParamMax=[]  IParamMin=[]  IParamMax=[]  DParamMin=[]  DParamMax=[]  NParamMin=[]  NParamMax=[]  KbParamMin=[]  KbParamMax=[]  KtParamMin=[]  KtParamMax=[]  KbOutMin=[]  KbOutMax=[]  KtOutMin=[]  KtOutMax=[]  IntegratorOutMin=[]  IntegratorOutMax=[]  FilterOutMin=[]  FilterOutMax=[]  SumI1OutMin=[]  SumI1OutMax=[]  SumI2OutMin=[]  SumI2OutMax=[]  SumI3OutMin=[]  SumI3OutMax=[]  SumI4OutMin=[]  SumI4OutMax=[]  SumDOutMin=[]  SumDOutMax=[]  DifferentiatorOutMin=[]  DifferentiatorOutMax=[]  FilterDiffOutCoefMin=[]  FilterDiffOutCoefMax=[]  ReciprocalOutMin=[]  ReciprocalOutMax=[]  SumDenOutMin=[]  SumDenOutMax=[]  SumNumOutMin=[]  SumNumOutMax=[]  DivideOutMin=[]  DivideOutMax=[]  UdiffTsProdOutMin=[]  UdiffTsProdOutMax=[]  NTsProdOutMin=[]  NTsProdOutMax=[]  UintegralTsProdOutMin=[]  UintegralTsProdOutMax=[]  UngainTsProdOutMin=[]  UngainTsProdOutMax=[]  IntegratorContinuousStateAttributes=''  IntegratorStateMustResolveToSignalObject=off  IntegratorRTWStateStorageClass=Auto  FilterContinuousStateAttributes=''  FilterStateMustResolveToSignalObject=off  FilterRTWStateStorageClass=Auto  ParallelPVariant=InternalParameters  IdealPVariant=Disabled  IVariant=InternalParameters  DVariant=Disabled  IntegratorVariant=Continuous  SatVariant=Disabled  AWVariant=Passthrough  PCopyVariant=Disabled  TRVariant=Disabled  FdbkBlocksVariant=Forward  IdealPFdbkVariant=Disabled  SatFdbkVariant=Disabled  DerivativeFilterVariant=Disabled  NVariant=Disabled  NCopyVariant=Disabled_SignalSpec  FilterICVariant=Disabled  IntegratorICVariant=InternalICs  ExternalResetVariant=Disabled  TRSumVariant=Passthrough  SumFdbkVariant=Disabled  SumVariant=Sum_PI  TsampFilterVariant=InternalTs  TsampNgainVariant=Passthrough  TsampIntegralVariant=Passthrough  ExternalSaturationOutDataTypeStr=Inherit: Same as second input  aMode=0
  PID Controller2 : slpidlib/PID Controller  Controller=PI  Form=Parallel  TimeDomain=Continuous-time  UseExternalTs=off  SampleTime=-1  IntegratorMethod=Forward Euler  FilterMethod=Forward Euler  ControllerParametersSource=internal  P=Kpi  I=Kii  UseKiTs=off  D=0  N=100  UseFilter=on  TunerSelectOption=Transfer Function Based (PID Tuner App)  InitialConditionSource=internal  InitialConditionForIntegrator=0  InitialConditionForFilter=0  DifferentiatorICPrevScaledInput=0  ExternalReset=none  TrackingMode=off  Kt=1  LimitOutput=off  SatLimitsSource=internal  UpperSaturationLimit=inf  LowerSaturationLimit=-inf  LinearizeAsGain=on  AntiWindupMode=none  Kb=1  POutMin=[]  POutMax=[]  IOutMin=[]  IOutMax=[]  DOutMin=[]  DOutMax=[]  NOutMin=[]  NOutMax=[]  SumOutMin=[]  SumOutMax=[]  SaturationOutMin=[]  SaturationOutMax=[]  PParamMin=[]  PParamMax=[]  IParamMin=[]  IParamMax=[]  DParamMin=[]  DParamMax=[]  NParamMin=[]  NParamMax=[]  KbParamMin=[]  KbParamMax=[]  KtParamMin=[]  KtParamMax=[]  KbOutMin=[]  KbOutMax=[]  KtOutMin=[]  KtOutMax=[]  IntegratorOutMin=[]  IntegratorOutMax=[]  FilterOutMin=[]  FilterOutMax=[]  SumI1OutMin=[]  SumI1OutMax=[]  SumI2OutMin=[]  SumI2OutMax=[]  SumI3OutMin=[]  SumI3OutMax=[]  SumI4OutMin=[]  SumI4OutMax=[]  SumDOutMin=[]  SumDOutMax=[]  DifferentiatorOutMin=[]  DifferentiatorOutMax=[]  FilterDiffOutCoefMin=[]  FilterDiffOutCoefMax=[]  ReciprocalOutMin=[]  ReciprocalOutMax=[]  SumDenOutMin=[]  SumDenOutMax=[]  SumNumOutMin=[]  SumNumOutMax=[]  DivideOutMin=[]  DivideOutMax=[]  UdiffTsProdOutMin=[]  UdiffTsProdOutMax=[]  NTsProdOutMin=[]  NTsProdOutMax=[]  UintegralTsProdOutMin=[]  UintegralTsProdOutMax=[]  UngainTsProdOutMin=[]  UngainTsProdOutMax=[]  IntegratorContinuousStateAttributes=''  IntegratorStateMustResolveToSignalObject=off  IntegratorRTWStateStorageClass=Auto  FilterContinuousStateAttributes=''  FilterStateMustResolveToSignalObject=off  FilterRTWStateStorageClass=Auto  ParallelPVariant=InternalParameters  IdealPVariant=Disabled  IVariant=InternalParameters  DVariant=Disabled  IntegratorVariant=Continuous  SatVariant=Disabled  AWVariant=Passthrough  PCopyVariant=Disabled  TRVariant=Disabled  FdbkBlocksVariant=Forward  IdealPFdbkVariant=Disabled  SatFdbkVariant=Disabled  DerivativeFilterVariant=Disabled  NVariant=Disabled  NCopyVariant=Disabled_SignalSpec  FilterICVariant=Disabled  IntegratorICVariant=InternalICs  ExternalResetVariant=Disabled  TRSumVariant=Passthrough  SumFdbkVariant=Disabled  SumVariant=Sum_PI  TsampFilterVariant=InternalTs  TsampNgainVariant=Passthrough  TsampIntegralVariant=Passthrough  ExternalSaturationOutDataTypeStr=Inherit: Same as second input  aMode=0
  PID Controller3 : slpidlib/PID Controller  Controller=PI  Form=Parallel  TimeDomain=Continuous-time  UseExternalTs=off  SampleTime=-1  IntegratorMethod=Forward Euler  FilterMethod=Forward Euler  ControllerParametersSource=internal  P=Kpi  I=Kii  UseKiTs=off  D=0  N=100  UseFilter=on  TunerSelectOption=Transfer Function Based (PID Tuner App)  InitialConditionSource=internal  InitialConditionForIntegrator=0  InitialConditionForFilter=0  DifferentiatorICPrevScaledInput=0  ExternalReset=none  TrackingMode=off  Kt=1  LimitOutput=off  SatLimitsSource=internal  UpperSaturationLimit=inf  LowerSaturationLimit=-inf  LinearizeAsGain=on  AntiWindupMode=none  Kb=1  POutMin=[]  POutMax=[]  IOutMin=[]  IOutMax=[]  DOutMin=[]  DOutMax=[]  NOutMin=[]  NOutMax=[]  SumOutMin=[]  SumOutMax=[]  SaturationOutMin=[]  SaturationOutMax=[]  PParamMin=[]  PParamMax=[]  IParamMin=[]  IParamMax=[]  DParamMin=[]  DParamMax=[]  NParamMin=[]  NParamMax=[]  KbParamMin=[]  KbParamMax=[]  KtParamMin=[]  KtParamMax=[]  KbOutMin=[]  KbOutMax=[]  KtOutMin=[]  KtOutMax=[]  IntegratorOutMin=[]  IntegratorOutMax=[]  FilterOutMin=[]  FilterOutMax=[]  SumI1OutMin=[]  SumI1OutMax=[]  SumI2OutMin=[]  SumI2OutMax=[]  SumI3OutMin=[]  SumI3OutMax=[]  SumI4OutMin=[]  SumI4OutMax=[]  SumDOutMin=[]  SumDOutMax=[]  DifferentiatorOutMin=[]  DifferentiatorOutMax=[]  FilterDiffOutCoefMin=[]  FilterDiffOutCoefMax=[]  ReciprocalOutMin=[]  ReciprocalOutMax=[]  SumDenOutMin=[]  SumDenOutMax=[]  SumNumOutMin=[]  SumNumOutMax=[]  DivideOutMin=[]  DivideOutMax=[]  UdiffTsProdOutMin=[]  UdiffTsProdOutMax=[]  NTsProdOutMin=[]  NTsProdOutMax=[]  UintegralTsProdOutMin=[]  UintegralTsProdOutMax=[]  UngainTsProdOutMin=[]  UngainTsProdOutMax=[]  IntegratorContinuousStateAttributes=''  IntegratorStateMustResolveToSignalObject=off  IntegratorRTWStateStorageClass=Auto  FilterContinuousStateAttributes=''  FilterStateMustResolveToSignalObject=off  FilterRTWStateStorageClass=Auto  ParallelPVariant=InternalParameters  IdealPVariant=Disabled  IVariant=InternalParameters  DVariant=Disabled  IntegratorVariant=Continuous  SatVariant=Disabled  AWVariant=Passthrough  PCopyVariant=Disabled  TRVariant=Disabled  FdbkBlocksVariant=Forward  IdealPFdbkVariant=Disabled  SatFdbkVariant=Disabled  DerivativeFilterVariant=Disabled  NVariant=Disabled  NCopyVariant=Disabled_SignalSpec  FilterICVariant=Disabled  IntegratorICVariant=InternalICs  ExternalResetVariant=Disabled  TRSumVariant=Passthrough  SumFdbkVariant=Disabled  SumVariant=Sum_PI  TsampFilterVariant=InternalTs  TsampNgainVariant=Passthrough  TsampIntegralVariant=Passthrough  ExternalSaturationOutDataTypeStr=Inherit: Same as second input  aMode=0
  Sum{,1,4..5} (4 alike) : Sum  Inputs=|+-
  Sum2 : Sum  Inputs=++-
  Sum3 : Sum  Inputs=+++
  Sum6 : Sum  Inputs=++-
  Sum7 : Sum  Inputs=+++
  dq0 to abc : spsdq0toabcLib/dq0 to abc  Alignment=90 degrees behind phase A axis
  UA : Outport
  UB : Outport  Port=2
  UC : Outport  Port=3
  wires:
  dq0 to abc/1 -> Demux/1
  PID Controller2/1 -> Sum6/2
  Vd/1 -> Sum6/1, Sum/2, Gain/1
  Demux/3 -> UC/1
  Gain3/1 -> Sum6/3
  id/1 -> Sum4/2, Gain2/1
  PID Controller1/1 -> Sum3/2
  Vdref/1 -> Sum/1
  Demux/1 -> UA/1
  Vqref/1 -> Sum1/1
  Sum4/1 -> PID Controller2/1
  Vq/1 -> Sum7/3, Gain1/1, Sum1/2
  Sum1/1 -> PID Controller1/1
  Gain2/1 -> Sum7/1
  Demux/2 -> UB/1
  Gain1/1 -> Sum2/3
  isq/1 -> Sum3/3
  iq/1 -> Sum5/2, Gain3/1
  Sum/1 -> PID Controller/1
  Sum2/1 -> Sum4/1  "idref"
  Mux/1 -> dq0 to abc/1
  PID Controller3/1 -> Sum7/2
  Sum5/1 -> PID Controller3/1
  Gain/1 -> Sum3/1
  Sum3/1 -> Sum5/1  "iqref"
  PID Controller/1 -> Sum2/2
  isd/1 -> Sum2/1
  Sum6/1 -> Mux/1  "idref"
  Sum7/1 -> Mux/2  "iqref"
  wt/1 -> dq0 to abc/2

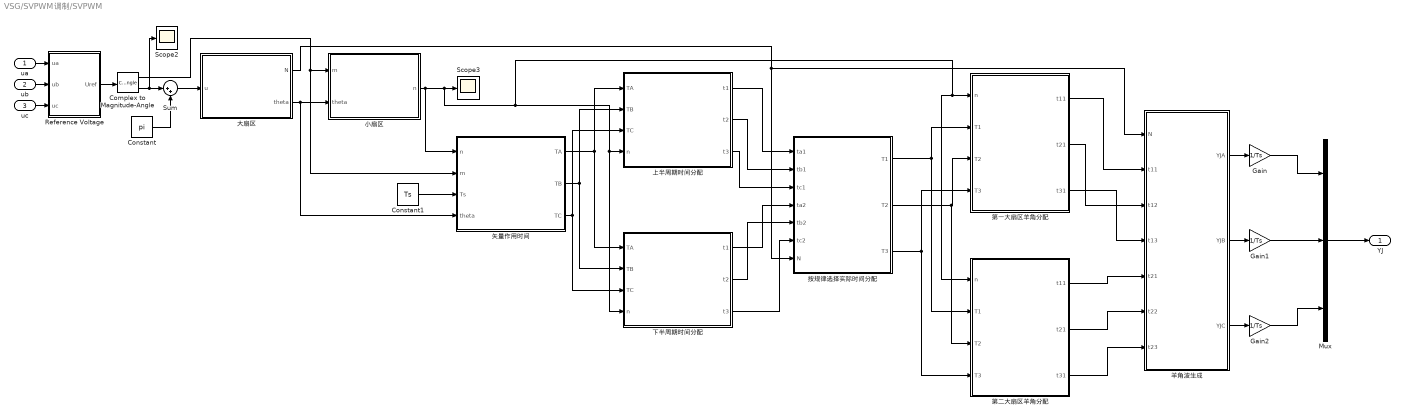
== system VSG/SVPWM调制/SVPWM ==
  ua : Inport
  ub : Inport  Port=2
  uc : Inport  Port=3
  Complex to Magnitude-Angle : ComplexToMagnitudeAngle
  Constant : Constant  Value=pi
  Constant1 : Constant  Value=Ts
  Gain : Gain  Gain=1/Ts
  Gain1 : Gain  Gain=1/Ts
  Gain2 : Gain  Gain=1/Ts
  Mux : Mux  Inputs=3
  Reference Voltage : MATLAB Function  TreatAsAtomicUnit=on
  Scope2 : Scope
  Scope3 : Scope
  Sum : Sum  Inputs=|++
  上半周期时间分配 : MATLAB Function  TreatAsAtomicUnit=on
  下半周期时间分配 : MATLAB Function  TreatAsAtomicUnit=on
  大扇区 : MATLAB Function  TreatAsAtomicUnit=on
  小扇区 : MATLAB Function  TreatAsAtomicUnit=on
  按规律选择实际时间分配 : MATLAB Function  TreatAsAtomicUnit=on
  矢量作用时间 : MATLAB Function  TreatAsAtomicUnit=on
  第一大扇区羊角分配 : MATLAB Function  TreatAsAtomicUnit=on
  第二大扇区羊角分配 : MATLAB Function  TreatAsAtomicUnit=on
  羊角波生成 : MATLAB Function  TreatAsAtomicUnit=on
  YJ : Outport
  wires:
  按规律选择实际时间分配/1(T1) -> 第二大扇区羊角分配/2(T1), 第一大扇区羊角分配/2(T1)
  Constant1/1 -> 矢量作用时间/3(Ts)
  Gain/1 -> Mux/1
  Sum/1 -> 大扇区/1(u)
  矢量作用时间/2(TB) -> 上半周期时间分配/2(TB), 下半周期时间分配/2(TB)
  按规律选择实际时间分配/3(T3) -> 第二大扇区羊角分配/4(T3), 第一大扇区羊角分配/4(T3)
  矢量作用时间/3(TC) -> 上半周期时间分配/3(TC), 下半周期时间分配/3(TC)
  小扇区/1(n) -> 第一大扇区羊角分配/1(n), 第二大扇区羊角分配/1(n), 下半周期时间分配/4(n), 上半周期时间分配/4(n), Scope3/1, 矢量作用时间/1(n)
  Reference Voltage/1(Uref) -> Complex to Magnitude-Angle/1
  Gain1/1 -> Mux/2
  上半周期时间分配/3(t3) -> 按规律选择实际时间分配/3(tc1)
  下半周期时间分配/2(t2) -> 按规律选择实际时间分配/5(tb2)
  下半周期时间分配/1(t1) -> 按规律选择实际时间分配/4(ta2)
  大扇区/1(N) -> 按规律选择实际时间分配/7(N), 羊角波生成/1(N)
  Constant/1 -> Sum/2
  上半周期时间分配/2(t2) -> 按规律选择实际时间分配/2(tb1)
  第二大扇区羊角分配/2(t21) -> 羊角波生成/6(t22)
  Complex to Magnitude-Angle/1 -> 矢量作用时间/2(m), 小扇区/1(m)
  大扇区/2(theta) -> 小扇区/2(theta), 矢量作用时间/4(theta)
  第一大扇区羊角分配/2(t21) -> 羊角波生成/3(t12)
  第一大扇区羊角分配/3(t31) -> 羊角波生成/4(t13)
  下半周期时间分配/3(t3) -> 按规律选择实际时间分配/6(tc2)
  第二大扇区羊角分配/1(t11) -> 羊角波生成/5(t21)
  ub/1 -> Reference Voltage/2(ub)
  Complex to Magnitude-Angle/2 -> Scope2/1, Sum/1
  羊角波生成/1(YJA) -> Gain/1
  第一大扇区羊角分配/1(t11) -> 羊角波生成/2(t11)
  上半周期时间分配/1(t1) -> 按规律选择实际时间分配/1(ta1)
  矢量作用时间/1(TA) -> 下半周期时间分配/1(TA), 上半周期时间分配/1(TA)
  羊角波生成/2(YJB) -> Gain1/1
  按规律选择实际时间分配/2(T2) -> 第二大扇区羊角分配/3(T2), 第一大扇区羊角分配/3(T2)
  羊角波生成/3(YJC) -> Gain2/1
  第二大扇区羊角分配/3(t31) -> 羊角波生成/7(t23)
  ua/1 -> Reference Voltage/1(ua)
  Mux/1 -> YJ/1
  Gain2/1 -> Mux/3
  uc/1 -> Reference Voltage/3(uc)

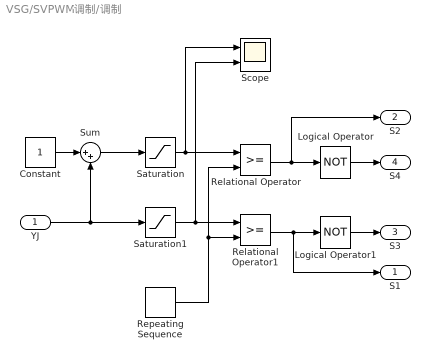
== system VSG/SVPWM调制/调制 ==
  YJ : Inport
  Constant : Constant
  Logical Operator : Logic  Operator=NOT  AllPortsSameDT=off  OutDataTypeStr=boolean
  Logical Operator1 : Logic  Operator=NOT  AllPortsSameDT=off  OutDataTypeStr=boolean
  Relational Operator : RelationalOperator  OutDataTypeStr=boolean  RndMeth=Simplest  InputSameDT=off
  Relational Operator1 : RelationalOperator  OutDataTypeStr=boolean  RndMeth=Simplest  InputSameDT=off
  Repeating Sequence : simulink/Sources/Repeating Sequence  rep_seq_t=[0 0.5*Ts Ts]  rep_seq_y=[1 0 1]
  Saturation : Saturate  UpperLimit=1  LowerLimit=0
  Saturation1 : Saturate  UpperLimit=1  LowerLimit=0
  Scope : Scope  NumInputPorts=2
  Sum : Sum  Inputs=|++
  S1 : Outport
  S2 : Outport  Port=2
  S3 : Outport  Port=3
  S4 : Outport  Port=4
  wires:
  Constant/1 -> Sum/1
  Relational Operator1/1 -> S1/1, Logical Operator1/1
  Saturation/1 -> Scope/1, Relational Operator/1
  YJ/1 -> Saturation1/1, Sum/2
  Relational Operator/1 -> S2/1, Logical Operator/1
  Logical Operator/1 -> S4/1
  Logical Operator1/1 -> S3/1
  Sum/1 -> Saturation/1
  Repeating Sequence/1 -> Relational Operator1/2, Relational Operator/2
  Saturation1/1 -> Scope/2, Relational Operator1/1

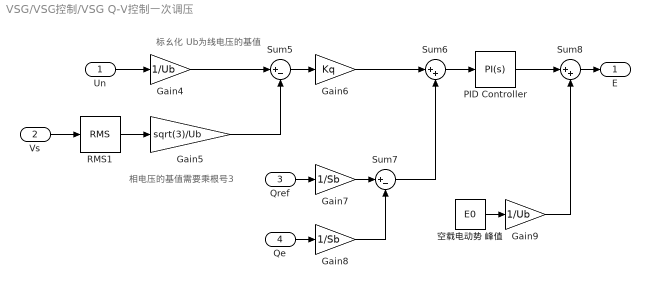
== system VSG/VSG控制/VSG Q-V控制一次调压 ==
  note: 标幺化 Ub为线电压的基值
  note: 相电压的基值需要乘根号3
  Un : Inport
  Vs : Inport  Port=2
  Qref : Inport  Port=3
  Qe : Inport  Port=4
  Gain4 : Gain  Gain=1/Ub
  Gain5 : Gain  Gain=sqrt(3)/Ub
  Gain6 : Gain  Gain=Kq
  Gain7 : Gain  Gain=1/Sb
  Gain8 : Gain  Gain=1/Sb
  Gain9 : Gain  Gain=1/Ub
  PID Controller : slpidlib/PID Controller  Controller=PI  Form=Parallel  TimeDomain=Continuous-time  UseExternalTs=off  SampleTime=-1  IntegratorMethod=Forward Euler  FilterMethod=Forward Euler  ControllerParametersSource=internal  P=0  I=Ki  UseKiTs=off  D=0  N=100  UseFilter=on  TunerSelectOption=Transfer Function Based (PID Tuner App)  InitialConditionSource=internal  InitialConditionForIntegrator=0  InitialConditionForFilter=0  DifferentiatorICPrevScaledInput=0  ExternalReset=none  TrackingMode=off  Kt=1  LimitOutput=off  SatLimitsSource=internal  UpperSaturationLimit=inf  LowerSaturationLimit=-inf  LinearizeAsGain=on  AntiWindupMode=none  Kb=1  POutMin=[]  POutMax=[]  IOutMin=[]  IOutMax=[]  DOutMin=[]  DOutMax=[]  NOutMin=[]  NOutMax=[]  SumOutMin=[]  SumOutMax=[]  SaturationOutMin=[]  SaturationOutMax=[]  PParamMin=[]  PParamMax=[]  IParamMin=[]  IParamMax=[]  DParamMin=[]  DParamMax=[]  NParamMin=[]  NParamMax=[]  KbParamMin=[]  KbParamMax=[]  KtParamMin=[]  KtParamMax=[]  KbOutMin=[]  KbOutMax=[]  KtOutMin=[]  KtOutMax=[]  IntegratorOutMin=[]  IntegratorOutMax=[]  FilterOutMin=[]  FilterOutMax=[]  SumI1OutMin=[]  SumI1OutMax=[]  SumI2OutMin=[]  SumI2OutMax=[]  SumI3OutMin=[]  SumI3OutMax=[]  SumI4OutMin=[]  SumI4OutMax=[]  SumDOutMin=[]  SumDOutMax=[]  DifferentiatorOutMin=[]  DifferentiatorOutMax=[]  FilterDiffOutCoefMin=[]  FilterDiffOutCoefMax=[]  ReciprocalOutMin=[]  ReciprocalOutMax=[]  SumDenOutMin=[]  SumDenOutMax=[]  SumNumOutMin=[]  SumNumOutMax=[]  DivideOutMin=[]  DivideOutMax=[]  UdiffTsProdOutMin=[]  UdiffTsProdOutMax=[]  NTsProdOutMin=[]  NTsProdOutMax=[]  UintegralTsProdOutMin=[]  UintegralTsProdOutMax=[]  UngainTsProdOutMin=[]  UngainTsProdOutMax=[]  IntegratorContinuousStateAttributes=''  IntegratorStateMustResolveToSignalObject=off  IntegratorRTWStateStorageClass=Auto  FilterContinuousStateAttributes=''  FilterStateMustResolveToSignalObject=off  FilterRTWStateStorageClass=Auto  ParallelPVariant=InternalParameters  IdealPVariant=Disabled  IVariant=InternalParameters  DVariant=Disabled  IntegratorVariant=Continuous  SatVariant=Disabled  AWVariant=Passthrough  PCopyVariant=Disabled  TRVariant=Disabled  FdbkBlocksVariant=Forward  IdealPFdbkVariant=Disabled  SatFdbkVariant=Disabled  DerivativeFilterVariant=Disabled  NVariant=Disabled  NCopyVariant=Disabled_SignalSpec  FilterICVariant=Disabled  IntegratorICVariant=InternalICs  ExternalResetVariant=Disabled  TRSumVariant=Passthrough  SumFdbkVariant=Disabled  SumVariant=Sum_PI  TsampFilterVariant=InternalTs  TsampNgainVariant=Passthrough  TsampIntegralVariant=Passthrough  ExternalSaturationOutDataTypeStr=Inherit: Same as second input  aMode=0
  RMS1 : dspstat3/RMS  run=off  directionMode=Each column  dimension=1  InputProcessing=Columns as channels (frame based)  reset_popup=None
  Sum5 : Sum  Inputs=|+-
  Sum6 : Sum  Inputs=|++
  Sum7 : Sum  Inputs=|+-
  Sum8 : Sum  Inputs=|++
  空载电动势 峰值 : Constant  Value=E0
  E : Outport
  wires:
  Un/1 -> Gain4/1
  Gain4/1 -> Sum5/1
  Vs/1 -> RMS1/1
  RMS1/1 -> Gain5/1
  Gain5/1 -> Sum5/2
  Sum5/1 -> Gain6/1
  Gain6/1 -> Sum6/1
  Qref/1 -> Gain7/1
  Qe/1 -> Gain8/1
  Gain7/1 -> Sum7/1
  Gain8/1 -> Sum7/2
  Sum7/1 -> Sum6/2
  Sum6/1 -> PID Controller/1
  PID Controller/1 -> Sum8/1
  空载电动势 峰值/1 -> Gain9/1
  Gain9/1 -> Sum8/2
  Sum8/1 -> E/1

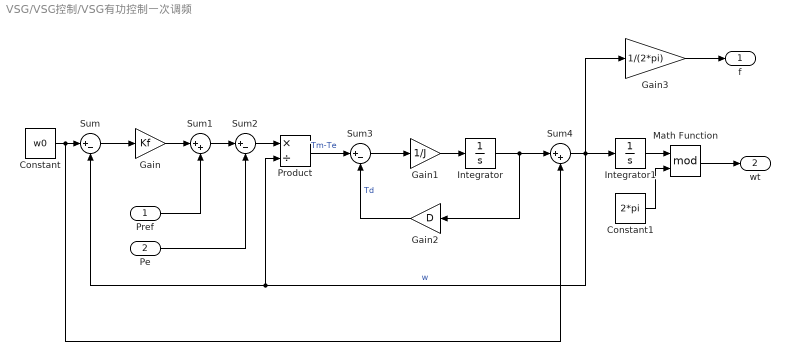
== system VSG/VSG控制/VSG有功控制一次调频 ==
  Pref : Inport
  Pe : Inport  Port=2
  Constant : Constant  Value=w0
  Constant1 : Constant  Value=2*pi
  Gain : Gain  Gain=Kf
  Gain1 : Gain  Gain=1/J
  Gain2 : Gain  Gain=D
  Gain3 : Gain  Gain=1/(2*pi)
  Integrator : Integrator
  Integrator1 : Integrator
  Math Function : Math  Operator=mod
  Product : Product  Inputs=*/
  Sum : Sum  Inputs=|+-
  Sum1 : Sum  Inputs=|++
  Sum2 : Sum  Inputs=|+-
  Sum3 : Sum  Inputs=|+-
  Sum4 : Sum  Inputs=|++
  f : Outport
  wt : Outport  Port=2
  wires:
  Pref/1 -> Sum1/2
  Sum4/1 -> Gain3/1, Product/2, Sum/2, Integrator1/1  "w"
  Constant/1 -> Sum4/2, Sum/1
  Gain1/1 -> Integrator/1
  Gain2/1 -> Sum3/2  "Td"
  Integrator/1 -> Sum4/1, Gain2/1
  Sum2/1 -> Product/1
  Product/1 -> Sum3/1  "Tm-Te"
  Sum/1 -> Gain/1
  Integrator1/1 -> Math Function/1
  Sum1/1 -> Sum2/1
  Math Function/1 -> wt/1
  Gain/1 -> Sum1/1
  Sum3/1 -> Gain1/1
  Pe/1 -> Sum2/2
  Gain3/1 -> f/1
  Constant1/1 -> Math Function/2

== matlab function VSG/SVPWM调制/SVPWM/第二大扇区羊角分配 ==
  data: n input; T1 input; T2 input; T3 input; t11 output; t21 output; t31 output
function [t11,t21,t31] = VectorShare(n,T1,T2,T3)
t11 = 0;
t21 = 0;
t31 = 0;
if (n==1)
    t11 = T1/2;
    t21 = T1/2+T3;
    t31 = -T1/2;
end
if (n==2)
    t11 = -T1/2;
    t21 = T1/2;
    t31 = -T1/2-T2;
end
if (n==3)
    t11 = T1/2;
    t21 = T1/2+T2+T3;
    t31 = -T1/2-T2;
end
if (n==4)
    t11 = -T1/2;
    t21 = T1/2+T3;
    t31 = -T1/2-T2-T3;
end
if (n==5)
    t11 = T1/2+T3;
    t21 = T1/2+T2+T3;
    t31 = -T1/2-T2-T3;
end
if (n==6)
    t11 = -T1/2-T2;
    t21 = T1/2+T2+T3;
    t31 = -T1/2-T2-T3;
end

== matlab function VSG/SVPWM调制/SVPWM/羊角波生成 ==
  data: N input; t11 input; t12 input; t13 input; YJA output; YJB output; YJC output; t21 input; t22 input; t23 input
function [YJA,YJB,YJC] = YangJiao(N,t11,t12,t13,t21,t22,t23)
YJA = 0;
YJB = 0;
YJC = 0;
if (N==1)
    YJA = t11;
    YJB = t12;
    YJC = t13;
end
if (N==2)
    YJA = t21;
    YJB = t22;
    YJC = t23;
end
if (N==3)
    YJA = t13;
    YJB = t11;
    YJC = t12;
end
if (N==4)
    YJA = t23;
    YJB = t21;
    YJC = t22;
end
if (N==5)
    YJA = t12;
    YJB = t13;
    YJC = t11;
end
if (N==6)
    YJA = t22;
    YJB = t23;
    YJC = t21;
end

== matlab function VSG/SVPWM调制/SVPWM/大扇区 ==
  data: u input; N output; theta output
function [N, theta] = BigVectorSwitch(u)

% Transfer to Section I
N = 0;
theta = 0;
thetaset = ceil(u/(pi/3));

u1 = u;
u2 = u-pi/3;
u3 = u-2*pi/3;
u4 = u-pi;
u5 = u-4*pi/3;
u6 = u-5*pi/3;

% Judge Section and Mapping
if (thetaset == 1)
    theta = u1;
    N = 4;
end

if (thetaset == 2)
    theta = u2;
    N = 5;
end

if (thetaset == 3)
    theta = u3;
    N = 6;
end

if (thetaset == 4)
    theta = u4;
    N = 1;
end

if (thetaset == 5)
    theta = u5;
    N = 2;
end

if (thetaset == 6)
    theta = u6;
    N = 3;
end

== matlab function VSG/SVPWM调制/SVPWM/Reference Voltage ==
  data: ua input; Uref output; ub input; uc input
function Uref = volt(ua,ub,uc)

Uref = (2/3) * (ua + ub*exp(1i*2*pi/3) + uc*exp(-1i*2*pi/3));

== matlab function VSG/SVPWM调制/SVPWM/小扇区 ==
  data: m input; n output; theta input
function n = SmallVectorSwitch(m, theta)

l_BD = -0.5 + m*sin(theta);
l_AB =  sqrt(3)*m*cos(theta) + m*sin(theta) -1;
l_AD = -sqrt(3)*m*cos(theta) + m*sin(theta) +1;

if (theta <= pi/6)
    if (l_AB <= 0)
        n=1;
    elseif (l_AD <= 0)
        n=5;
    else
        n=3;
    end
else
    if (l_AB <= 0)
        n=2;
    elseif (l_BD >= 0)
        n=6;
    else
        n=4;
    end
end

== matlab function VSG/SVPWM调制/SVPWM/矢量作用时间 ==
  data: n input; m input; Ts input; TA output; theta input; TB output; TC output
function [TA,TB,TC] = VectorTime(n,m,Ts,theta)

TA=0;
TB=0;
TC=0;

if (n==1 || n==2)
    TA = 2*m*Ts*sin(theta);
    TB = Ts*(1-2*m*sin(theta+pi/3));
    TC = 2*m*Ts*sin(-theta+pi/3);
end

if (n==3 || n==4)
    TA = Ts*(1-2*m*sin(theta));
    TB = Ts*(2*m*sin(pi/3+theta)-1);
    TC = Ts*(1-2*m*sin(pi/3-theta));
end

if (n==5)
    TA = 2*m*Ts*sin(theta);
    TB = 2*Ts*(1-m*sin(pi/3 + theta));
    TC = Ts*(2*m*sin(pi/3-theta)-1);
end

if (n==6)
    TA = Ts*(2*m*sin(theta)-1);
    TB = 2*Ts*(1-m*sin(pi/3 + theta));
    TC = 2*m*Ts*sin(pi/3-theta);
end

== matlab function VSG/SVPWM调制/SVPWM/上半周期时间分配 ==
  data: TA input; TB input; TC input; n input; t1 output; t2 output; t3 output
function [t1,t2,t3] = TimeShare(TA,TB,TC,n)

t1=0;
t2=0;
t3=0;

if (n==1)
    t1 = TC;
    t2 = TA;
    t3 = TB;
end

if (n==2)
    t1 = TA;
    t2 = TB;
    t3 = TC;
end

if (n==3)
    t1 = TA;
    t2 = TC;
    t3 = TB;
end

if (n==4)
    t1 = TC;
    t2 = TB;
    t3 = TA;
end

if (n==5)
    t1 = TB;
    t2 = TC;
    t3 = TA;
end

if (n==6)
    t1 = TB;
    t2 = TC;
    t3 = TA;
end
